simulink model "pi_test_2"  (R2021a)
settings: Solver=ode4  StartTime=0.0  StopTime=inf  FixedStep=0.001  RelTol=1e-3  EnableMultiTasking=on
undefined symbols (not defined in the file): k, z
libraries: arduinolib x4
settings Model: ExtModeTrigDuration=2  Creator=lcauf  LastModifiedBy=carol
settings SolverCC: AlgebraicLoopSolver=TrustRegion
settings OptimizationCC: EnhancedBackFolding=on  PassReuseOutputArgsThreshold=0  MaxStackSize=64  OptimizeBlockOrder=speed  DifferentSizesBufferReuse=on  OptimizationCustomize=off
settings DebuggingCC: ParameterTunabilityLossMsg=error
settings HardwareCC: ProdBitPerPointer=32  ProdBitPerSizeT=32  ProdBitPerPtrDiffT=32  ProdLargestAtomicInteger=Long  ProdLargestAtomicFloat=Double  ProdWordSize=32  ProdHWDeviceType=ARM Compatible->ARM Cortex  UseEmbeddedCoderFeatures=off  UseSimulinkCoderFeatures=off
settings SFSimCC: MATLABDynamicMemAlloc=off  CustomCodeUndefinedFunction=UseInterfaceOnly
settings RTWCC: SystemTargetFile=ert.tlc  HardwareBoard=Arduino Due  TemplateMakefile=ert_default_tmf  Toolchain=Arduino ARM  BuildConfiguration=Faster Runs
settings CodeAppCC: ForceParamTrailComments=on  OperatorAnnotations=on
settings ERTTargetCC: ERTCustomFileBanners=off  SupportContinuousTime=on  SupportNonInlinedSFcns=on  RemoveResetFunc=off  SupportVariableSizeSignals=on  ModelStepFunctionPrototypeControlCompliant=off  ExtMode=on  ExtModeTransport=3  ExtModeStaticAlloc=on  ExtModeStaticAllocSize=24576  ExtModeMexFile=ext_xcp  ExtModeMexArgs=0 3 115200 'C:\Users\Public\Downloads\validacao_arduino.elf' 3 1000  ExtModeIntrfLevel=Level2 - Open  ERTSrcFileBannerTemplate=codertarget_code_template.cgt  ERTHdrFileBannerTemplate=codertarget_code_template.cgt  ERTDataSrcFileTemplate=codertarget_code_template.cgt  ERTDataHdrFileTemplate=codertarget_code_template.cgt

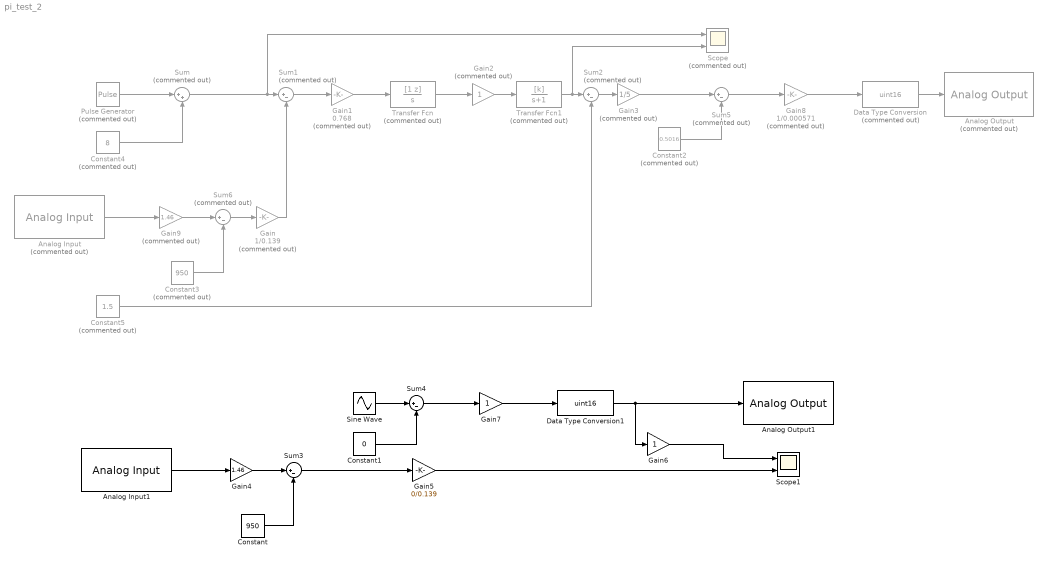
== system pi_test_2 ==
  Analog Input : arduinolib/Analog Input  Commented=on  pinNumber=0  ReadResultsOnly=off  ConversionTriggerSource=Software  ExternalTriggerType=uint32( 0 )  OutputDataType=uint16  EnableConversionCompleteNotify=off  EnableOuputStatus=off  SampleTime=-1  blockPlatform=arduino
  Analog Input1 : arduinolib/Analog Input  pinNumber=0  ReadResultsOnly=off  ConversionTriggerSource=Software  ExternalTriggerType=uint32( 0 )  OutputDataType=uint16  EnableConversionCompleteNotify=off  EnableOuputStatus=off  SampleTime=-1  blockPlatform=arduino
  Analog Output : arduinolib/Analog Output  Commented=on  DACpin=DAC0  blockPlatform=arduino
      settings: SourceProductBaseCode=ARDUINO
  Analog Output1 : arduinolib/Analog Output  DACpin=DAC0  blockPlatform=arduino
      settings: SourceProductBaseCode=ARDUINO
  Constant : Constant  Value=950
  Constant1 : Constant  Value=0
  Constant2 : Constant  Commented=on  Value=0.5016
  Constant3 : Constant  Commented=on  Value=950
  Constant4 : Constant  Commented=on  Value=8
  Constant5 : Constant  Commented=on  Value=1.5
  Data Type Conversion : DataTypeConversion  Commented=on  OutDataTypeStr=uint16
  Data Type Conversion1 : DataTypeConversion  OutDataTypeStr=uint16
  Gain : Gain  Commented=on  Gain=1/0.139
  Gain1 : Gain  Commented=on  Gain=0.768
  Gain2 : Gain  Commented=on
  Gain3 : Gain  Commented=on  Gain=1/5
  Gain4 : Gain  Gain=1.46
  Gain5 : Gain  Gain=0/0.139
  Gain6 : Gain
  Gain7 : Gain
  Gain8 : Gain  Commented=on  Gain=1/0.000571
  Gain9 : Gain  Commented=on  Gain=1.46
  Pulse Generator : DiscretePulseGenerator  Commented=on  PulseType=Time based  Amplitude=7  Period=3.33  PulseWidth=50
  Scope : Scope  Commented=on  NumInputPorts=2
  Scope1 : Scope  NumInputPorts=2
  Sine Wave : Sin  Amplitude=1550  Bias=1950  SampleTime=0
  Sum : Sum  Commented=on  Inputs=|++
  Sum{1..2,5..6} (4 alike) : Sum  Commented=on  Inputs=|+-
  Sum3 : Sum  Inputs=|+-
  Sum4 : Sum  Inputs=|+-
  Transfer Fcn : TransferFcn  Commented=on  Numerator=[1 z]  Denominator=[1 0]
  Transfer Fcn1 : TransferFcn  Commented=on  Numerator=[k]  Denominator=[1 1]
  wires:
  Data Type Conversion/1 -> Analog Output/1
  Pulse Generator/1 -> Sum/1
  Constant4/1 -> Sum/2
  Sum/1 -> Scope/1, Sum1/1
  Gain/1 -> Sum1/2
  Sum1/1 -> Gain1/1
  Transfer Fcn/1 -> Gain2/1
  Gain2/1 -> Transfer Fcn1/1
  Sum2/1 -> Gain3/1
  Transfer Fcn1/1 -> Scope/2, Sum2/1
  Constant5/1 -> Sum2/2
  Gain1/1 -> Transfer Fcn/1
  Data Type Conversion1/1 -> Gain6/1, Analog Output1/1
  Analog Input1/1 -> Gain4/1
  Gain4/1 -> Sum3/1
  Constant/1 -> Sum3/2
  Sum3/1 -> Gain5/1
  Gain5/1 -> Scope1/2
  Gain6/1 -> Scope1/1
  Gain7/1 -> Data Type Conversion1/1
  Sine Wave/1 -> Sum4/1
  Sum4/1 -> Gain7/1
  Constant1/1 -> Sum4/2
  Gain3/1 -> Sum5/1
  Sum5/1 -> Gain8/1
  Gain8/1 -> Data Type Conversion/1
  Constant2/1 -> Sum5/2
  Analog Input/1 -> Gain9/1
  Constant3/1 -> Sum6/2
  Gain9/1 -> Sum6/1
  Sum6/1 -> Gain/1
